simulink model "Parameter_Estimation_SM_Model"  (R2023b)
settings: Solver=VariableStepAuto  StartTime=0.0  StopTime=550  RelTol=1e-3
values from neighbouring files (symbols this model uses):
  D = 0.10692    [initial_consts.m]
  Gear_Ratio = 1    [initial_consts.m]
  J = 0.054058    [initial_consts.m]
  Kb = 0.68378    [initial_consts.m]
  Kt = 4.1772    [initial_consts.m]
  L = 0.00026447    [initial_consts.m]
  R = 0.067034    [initial_consts.m]
undefined symbols (not defined in the file or in its folder): sigbuilder_block
settings Model: Creator=Ahmed  LastModifiedBy=Ahmed
settings SolverCC: AlgebraicLoopSolver=TrustRegion
settings DebuggingCC: UnconnectedInputMsg=warning  UnconnectedOutputMsg=warning  UnconnectedLineMsg=warning
settings ModelReferenceCC: EnableRefExpFcnMdlSchedulingChecks=on

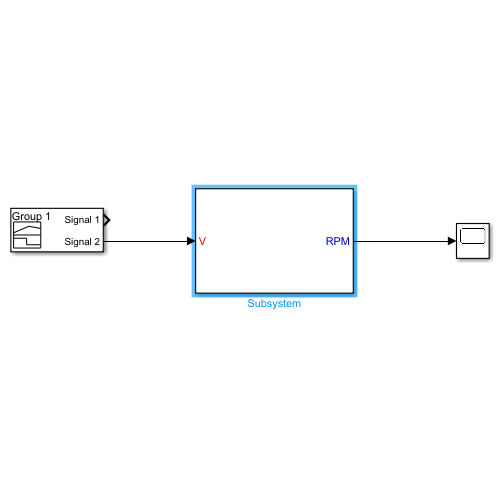
[thumbnail: Simulink's stored preview of the top-level diagram]
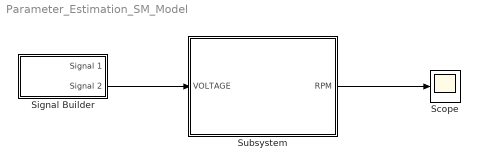
== system Parameter_Estimation_SM_Model ==
  Scope : Scope
  Signal Builder : Subsystem  Tag=STV Subsys  LoadFcn=sigbuilder_block('load');  StartFcn=sigbuilder_block('start');  StopFcn=sigbuilder_block('stop');  ClipboardFcn=sigbuilder_block('clipboard');  mask(Sigbuilder block){tuvar=[0:10]}
      mask help: Simulink:masks:SigbuilderBlock_MD
      mask init:
      | if ~strcmp(get_param(bdroot(gcbh),'SimulationStatus'),'stopped') tuvar = sigbuilder_block('maskInit'); end
      settings: CopyFcn=sigbuilder_block('copy');  DeleteFcn=sigbuilder_block('delete');  ModelCloseFcn=sigbuilder_block('modelClose');  PreSaveFcn=sigbuilder_block('preSave');  PauseFcn=sigbuilder_block('pause');  ContinueFcn=sigbuilder_block('continue');  NameChangeFcn=sigbuilder_block('namechange');  OpenFcn=sigbuilder_block('open',[251.25 72.75 550.5 417.75 ]);  CloseFcn=sigbuilder_block('close');
      mask Display: plot(0, 0, 100, 100,[2, 2, 32, 32, 2], [68, 8, 8, 68, 68],[32, 2], [38, 38], [32, 19, 2],[53, 60, 44], [32, 17, 17, 2],[16, 16, 31, 31]);txt = getActiveGroup(gcbh);text(2, 100, txt,'verticalAlignment', 'top');
  Subsystem : Subsystem
      mask Display:
      | color ('red')
      | port_label('input',1,'V')
      | color ('blue')
      | port_label('output',1,'RPM')
  wires:
  Subsystem/1(RPM) -> Scope/1
  Signal Builder/2(Signal 2) -> Subsystem/1(VOLTAGE)

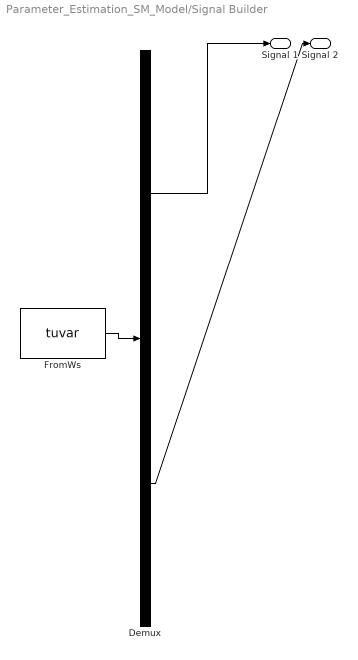
== system Parameter_Estimation_SM_Model/Signal Builder ==
  Demux : Demux  Tag=STV Demux  Outputs=2
      settings: DisplayOption=none
  FromWs : FromWorkspace  Tag=STV FromWs  VariableName=tuvar
      SigBuilderData=|
      | common.afterFinalStr = 'Extrapolate'
      | common.sampleTime = 0
      | dataSet.timeRange = [0 550]
      | dataSet.name = 'Group 1'
      | sbobj.Groups.Name = 'Group 1'
      | sbobj.Groups.Signals(1).Name = 'Signal 1'
      | sbobj.Groups.Signals(1).XData = [0 0.1 0.2 0.3 0.4 0.5 0.6 0.7 0.8 0.9 1 1.1 ... (1452 elements, 1x1452)]
      | sbobj.Groups.Signals(1).YData = [0 0 0 0 0 0 0 -0.2 -0.2 -0.2 -0.2 -0.2 ... (1452 elements, 1x1452)]
      | sbobj.Groups.Signals(2).Name = 'Signal 2'
      | sbobj.Groups.Signals(2).XData = [0 0.1 0.2 0.3 0.4 0.5 0.6 0.7 0.8 0.9 1 1.1 ... (5244 elements, 1x5244)]
      | sbobj.Groups.Signals(2).YData = [-0.39 -0.39 -0.39 -0.39 -0.39 -0.39 -0.39 -0.39 -0.39 -0.39 -0.39 -0.39 ... (5244 elements, 1x5244)]
      | sbobj.Groups.TimeRange = [0 550]
  Signal 1 : Outport  Tag=STV Outport
  Signal 2 : Outport  Tag=STV Outport  Port=2
  wires:
  FromWs/1 -> Demux/1
  Demux/1 -> Signal 1/1
  Demux/2 -> Signal 2/1

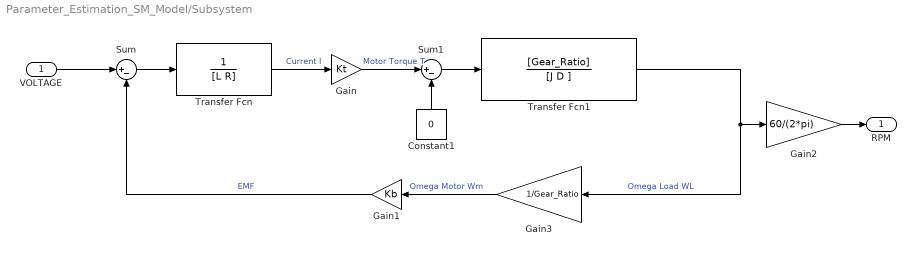
== system Parameter_Estimation_SM_Model/Subsystem ==
  VOLTAGE : Inport
  Constant1 : Constant  Value=0
  Gain : Gain  Gain=Kt
  Gain1 : Gain  Gain=Kb
  Gain2 : Gain  Gain=60/(2*pi)
  Gain3 : Gain  Gain=1/Gear_Ratio
  Sum : Sum  Inputs=|+-
  Sum1 : Sum  Inputs=|+-
  Transfer Fcn : TransferFcn  Denominator=[L R]
  Transfer Fcn1 : TransferFcn  Numerator=[Gear_Ratio]  Denominator=[J D ]
  RPM : Outport
  wires:
  Transfer Fcn1/1 -> Gain2/1, Gain3/1  "Omega Load WL"
  Transfer Fcn/1 -> Gain/1  "Current I"
  Gain/1 -> Sum1/1  "Motor Torque T"
  Sum/1 -> Transfer Fcn/1
  Sum1/1 -> Transfer Fcn1/1
  Constant1/1 -> Sum1/2
  Gain1/1 -> Sum/2  "EMF"
  VOLTAGE/1 -> Sum/1
  Gain2/1 -> RPM/1
  Gain3/1 -> Gain1/1  "Omega Motor Wm"
